simulink library "Desaturation_Controller_lib_old"  (R2018b)
settings: Solver=VariableStepAuto  StartTime=0.0  StopTime=10.0  RelTol=1e-3
undefined symbols (not defined in the file or in its folder): fswParams
libraries: vrlib x1
settings Model: Creator=colem  LastModifiedBy=colem

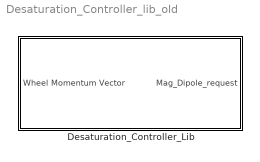
== system Desaturation_Controller_lib_old ==
  Desaturation_Controller_Lib : Subsystem

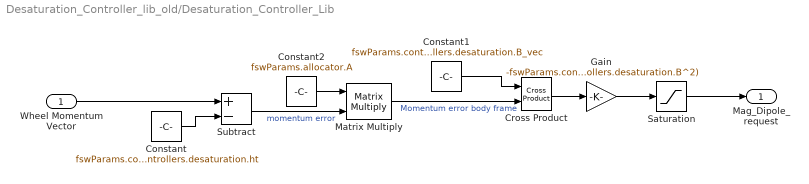
== system Desaturation_Controller_lib_old/Desaturation_Controller_Lib ==
  Wheel Momentum Vector : Inport
  Constant : Constant  Value=fswParams.controllers.desaturation.ht
  Constant1 : Constant  Value=fswParams.controllers.desaturation.B_vec
  Constant2 : Constant  Value=fswParams.allocator.A
  Cross Product : vrlib/Utilities/Cross Product
      settings: SourceProductBaseCode=VR
  Gain : Gain  Gain=-fswParams.controllers.desaturation.k/(fswParams.controllers.desaturation.B^2)
  Matrix Multiply : Product  Multiplication=Matrix(*)
  Saturation : Saturate  UpperLimit=fswParams.controllers.desaturation.maxDipole  LowerLimit=-fswParams.controllers.desaturation.maxDipole
  Subtract : Sum  Inputs=+-
  Mag_Dipole_request : Outport
  wires:
  Constant/1 -> Subtract/2
  Constant2/1 -> Matrix Multiply/1
  Constant1/1 -> Cross Product/1
  Matrix Multiply/1 -> Cross Product/2  "Momentum error body frame"
  Subtract/1 -> Matrix Multiply/2  "momentum error"
  Cross Product/1 -> Gain/1
  Wheel Momentum Vector/1 -> Subtract/1
  Gain/1 -> Saturation/1
  Saturation/1 -> Mag_Dipole_request/1
